simulink model "Main"  (Simulink 7.9)
settings: Solver=ode4  StartTime=0.0  StopTime=inf  RelTol=1e-3
libraries: simulink x1, rtweclib x1, commfilt2 x1, idelinklib_tgtpref x1
settings Model: Creator=spacekitteh  LastModifiedBy=spacekitteh
settings SolverCC: PositivePriorityOrder=on
settings DataIOCC: SaveOutput=off  SaveTime=off
settings OptimizationCC: InlineParams=on  InlineInvariantSignals=on  StateBitsets=on  DataBitsets=on  UseTempVars=on  ZeroExternalMemoryAtStartup=off  NoFixptDivByZeroProtection=on  EfficientFloat2IntCast=on  OptimizeModelRefInitCode=on  LifeSpan=1  SimCompilerOptimization=On
settings HardwareCC: ProdLargestAtomicInteger=Long  ProdLargestAtomicFloat=Double  ProdIntDivRoundTo=Zero  ProdEndianess=LittleEndian  ProdHWDeviceType=ARMCortex  TargetLargestAtomicInteger=Long  TargetLargestAtomicFloat=Double  TargetIntDivRoundTo=Zero  TargetEndianess=LittleEndian  TargetHWDeviceType=ARM Compatible->ARM Cortex  ProdEqTarget=off
settings RTWCC: SystemTargetFile=ert.tlc  GenCodeOnly=on  TemplateMakefile=ert_default_tmf  Description=Embedded Coder  GenerateReport=on  RTWVerbose=off  ProcessScript=ert_make_rtw_hook  IncludeHyperlinkInReport=on  LaunchReport=on  TargetLang=C++  GenerateTraceInfo=on  GenerateTraceReport=on  GenerateTraceReportSl=on  GenerateTraceReportSf=on  GenerateTraceReportEml=on
settings CodeAppCC: ForceParamTrailComments=on  IgnoreCustomStorageClasses=off  SimulinkDataObjDesc=on  CustomSymbolStrGlobalVar=rt$N$M  CustomSymbolStrType=$N$M  CustomSymbolStrFcn=$N$M$F  CustomSymbolStrMacro=$N$M  InsertBlockDesc=on
settings ERTTargetCC: CodeReplacementLibrary=GCC ARM Cortex-A8  MultiwordLength=2048  GenerateSampleERTMain=on  CombineOutputUpdateFcns=off  MultiInstanceERTCode=on  SupportContinuousTime=on  InlinedParameterPlacement=NonHierarchical  ERTCustomFileTemplate=example_file_process.tlc  ConvertIfToSwitch=off  SuppressUnreachableDefaultCases=off

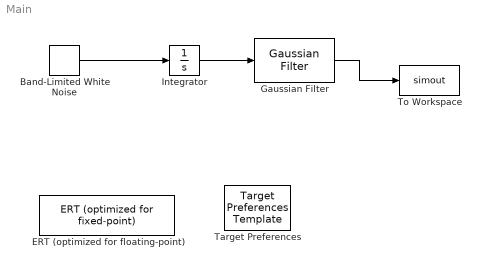
== system Main ==
  Band-Limited White Noise : simulink/Sources/Band-Limited White Noise  Cov=[0.1 0.1 0.1]  Ts=0.1  seed=[23341]
  ERT (optimized for floating-point) : rtweclib/Configuration Wizards/ERT (optimized for fixed-point)  ConfigMode=ERT (optimized for floating-point)  ConfigScript=rtwsampleconfig  InvokeBuild=off  ShowInLibBrowser=off
  Gaussian Filter : commfilt2/Gaussian Filter  N=8  BT=0.3  D=2  sampMode=Frame-based  normMode=Sum of coefficients  filterGain=1  checkCoeff=off  variableName=gaussFilt  launchFVT=off  roundingMode=Floor  overflowMode=off  InputProcessing=Columns as channels (frame based)
  Integrator : Integrator
  Target Preferences : idelinklib_tgtpref/Target Preferences Template  Tag=eclipseidetgtpref  library=off
  To Workspace : ToWorkspace  VariableName=simout  SampleTime=-1  SaveFormat=Timeseries
  wires:
  Band-Limited White Noise/1 -> Integrator/1
  Integrator/1 -> Gaussian Filter/1
  Gaussian Filter/1 -> To Workspace/1
